simulink model "model2"  (R2024b)
settings: Solver=VariableStepAuto  StartTime=0.0  StopTime=5  MaxStep=1e-3  RelTol=1e-3
values from neighbouring files (symbols this model uses):
  A = -1    [run.m]    (also in temp.m; test.m)
  Bw = 1    [run.m]    (also in temp.m; test.m)
  C0 = [1;2]    [run.m]    (also in temp.m; test.m)
  Ctheta = [1;0]    [run.m]    (also in temp.m = H*[1;1+1e-2]*E)
  Dw = [1;2]*1+[2;-1]*1    [run.m]    (also in temp.m; test.m)
  L = inv(P)*Y    [run.m]    (also in test.m = [20,20])
  Pi0 = eye(p)-C0*pinv(C0'*C0)*C0'    [run.m]    (also in temp.m = proj(C0); test.m = proj(C0))
  theta_test = 0.5    [run.m]
settings Model: Creator=Mehmet  LastModifiedBy=Mehmet

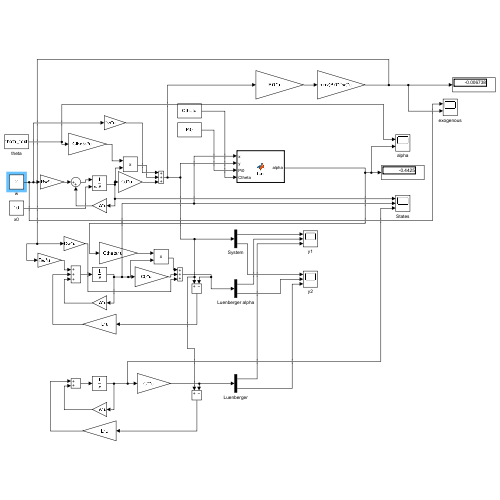
[thumbnail: Simulink's stored preview of the top-level diagram]
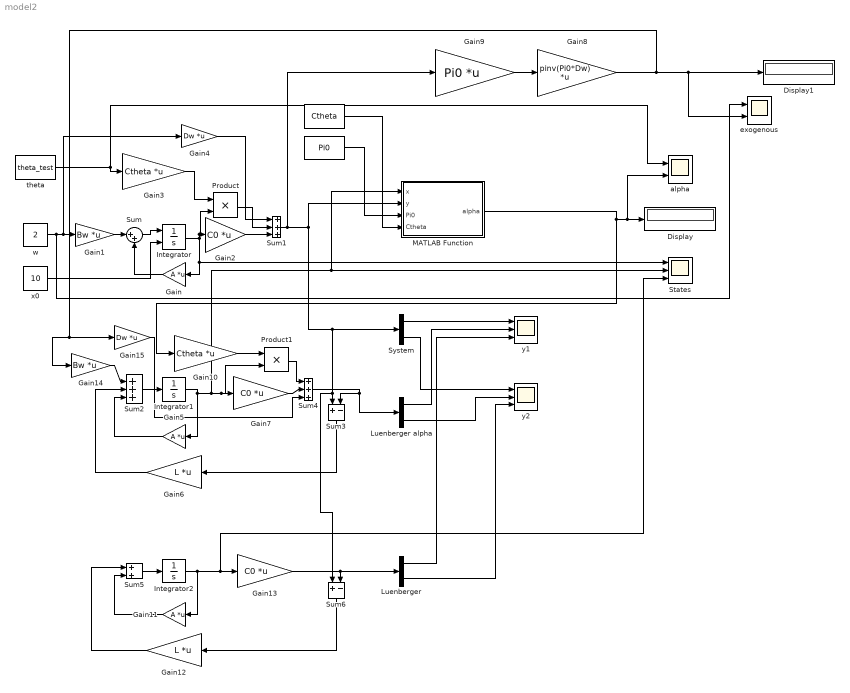
== system model2 ==
  " " : Constant  Value=Pi0
  "  " : Constant  Value=Ctheta
  Display : Display
  Display1 : Display
  Gain : Gain  Gain=A  Multiplication=Matrix(K*u)
  Gain1 : Gain  Gain=Bw  Multiplication=Matrix(K*u)
  Gain10 : Gain  Gain=Ctheta  Multiplication=Matrix(K*u)
  Gain11 : Gain  Gain=A  Multiplication=Matrix(K*u)
  Gain12 : Gain  Gain=L  Multiplication=Matrix(K*u)
  Gain13 : Gain  Gain=C0  Multiplication=Matrix(K*u)
  Gain14 : Gain  Gain=Bw  Multiplication=Matrix(K*u)
  Gain15 : Gain  Gain=Dw  Multiplication=Matrix(K*u)
  Gain2 : Gain  Gain=C0  Multiplication=Matrix(K*u)
  Gain3 : Gain  Gain=Ctheta  Multiplication=Matrix(K*u)
  Gain4 : Gain  Gain=Dw  Multiplication=Matrix(K*u)
  Gain5 : Gain  Gain=A  Multiplication=Matrix(K*u)
  Gain6 : Gain  Gain=L  Multiplication=Matrix(K*u)
  Gain7 : Gain  Gain=C0  Multiplication=Matrix(K*u)
  Gain8 : Gain  Gain=pinv(Pi0*Dw)  Multiplication=Matrix(K*u)
  Gain9 : Gain  Gain=Pi0  Multiplication=Matrix(K*u)
  Integrator : Integrator  InitialConditionSource=external
  Integrator1 : Integrator
  Integrator2 : Integrator
  Luenberger : Demux  Outputs=2
  Luenberger alpha : Demux  Outputs=2
  MATLAB Function : MATLAB Function  TreatAsAtomicUnit=on
  Product : Product
  Product1 : Product
  States : Scope  NumInputPorts=3
  Sum : Sum  Inputs=|++
  Sum1 : Sum  Inputs=+++
  Sum2 : Sum  Inputs=+++
  Sum3 : Sum  Inputs=+-
  Sum4 : Sum  Inputs=+++
  Sum5 : Sum
  Sum6 : Sum  Inputs=+-
  System : Demux  Outputs=2
  alpha : Scope  NumInputPorts=2
  exogenous : Scope  NumInputPorts=2
  theta : Constant  Value=theta_test
  w : Constant  Value=2
  x0 : Constant  Value=10
  y1 : Scope  NumInputPorts=3
  y2 : Scope  NumInputPorts=3
  wires:
  Integrator/1 -> Product/2, Gain2/1, Gain/1, States/1
  Sum/1 -> Integrator/1
  Gain/1 -> Sum/2
  Gain1/1 -> Sum/1
  w/1 -> exogenous/1, Gain4/1, Gain1/1
  theta/1 -> Gain3/1, alpha/1
  Gain2/1 -> Sum1/3
  Gain3/1 -> Product/1
  Gain4/1 -> Sum1/1
  x0/1 -> Integrator/2
  Integrator1/1 -> Product1/2, Gain7/1, States/2, MATLAB Function/1(x), Gain5/1
  Sum2/1 -> Integrator1/1
  Gain5/1 -> Sum2/3
  Gain6/1 -> Sum2/2
  Sum1/1 -> Gain9/1, Sum6/1, Sum3/1, System/1, MATLAB Function/2(y)
  System/1 -> y1/1
  System/2 -> y2/1
  Sum4/1 -> Sum3/2, Luenberger alpha/1
  Sum3/1 -> Gain6/1
  Luenberger alpha/1 -> y1/2
  Luenberger alpha/2 -> y2/2
  Product/1 -> Sum1/2
  MATLAB Function/1(alpha) -> Gain10/1, Display/1, alpha/2
  Gain10/1 -> Product1/1
  Gain7/1 -> Sum4/2
  Product1/1 -> Sum4/1
  Gain12/1 -> Sum5/1
  Integrator2/1 -> States/3, Gain13/1, Gain11/1
  Gain11/1 -> Sum5/2
  Sum5/1 -> Integrator2/1
  Sum6/1 -> Gain12/1
  Gain13/1 -> Luenberger/1, Sum6/2
  Luenberger/1 -> y1/3
  Luenberger/2 -> y2/3
  " "/1 -> MATLAB Function/3(Pi0)
  "  "/1 -> MATLAB Function/4(Ctheta)
  Gain9/1 -> Gain8/1
  Gain8/1 -> Gain15/1, Gain14/1, Display1/1, exogenous/2
  Gain14/1 -> Sum2/1
  Gain15/1 -> Sum4/3

== matlab function model2/MATLAB Function ==
  data: x input; alpha output; y input; Pi0 input; Ctheta input
function alpha = fcn(x,y,Pi0,Ctheta)
    if abs(x)>=1e-2
        alpha=pinv(Pi0*Ctheta)*Pi0*y/x;
        if alpha>1
            alpha=1;
        elseif alpha<-1
            alpha=-1;
        end
    else
        alpha=0;
    end
end
